simulink model "hyun_PotensionMetor_To_Dcmotor"  (R2022b)
settings: Solver=ode4  StartTime=0.0  StopTime=inf  RelTol=1e-3  EnableMultiTasking=on
libraries: arduinolib x3
settings Model: ExtModeTrigDuration=2  Creator=user  LastModifiedBy=현대오토18
settings OptimizationCC: EnhancedBackFolding=on  PassReuseOutputArgsAs=Individual arguments  ZeroExternalMemoryAtStartup=off  ZeroInternalMemoryAtStartup=off  MaxStackSize=64  OptimizeBlockOrder=speed  DifferentSizesBufferReuse=on  OptimizationCustomize=off  EfficientTunableParamExpr=on
settings DebuggingCC: ParameterTunabilityLossMsg=error
settings HardwareCC: ProdBitPerInt=16  ProdBitPerPointer=16  ProdBitPerSizeT=16  ProdBitPerPtrDiffT=16  ProdLargestAtomicFloat=None  ProdWordSize=8  ProdHWDeviceType=Atmel->AVR
settings SFSimCC: MATLABDynamicMemAlloc=off
settings RTWCC: Description=Embedded Coder  SystemTargetFile=ert.tlc  HardwareBoard=Arduino Mega 2560  TLCOptions=-aInlineSetEventsForThisBaseRateFcn=TLC_FALSE -aSuppressMultiTaskScheduler=TLC_FALSE -aRateBasedStepFcn=1  TemplateMakefile=ert_default_tmf  Toolchain=Arduino AVR  BuildConfiguration=Faster Runs
settings CodeAppCC: ForceParamTrailComments=on  IgnoreCustomStorageClasses=off  OperatorAnnotations=on  SimulinkDataObjDesc=on  SFDataObjDesc=on  InsertBlockDesc=on
settings ERTTargetCC: SupportContinuousTime=on  SupportVariableSizeSignals=on  ExtModeTransport=3  ExtModeStaticAlloc=on  ExtModeAutomaticAllocSize=off  ExtModeStaticAllocSize=2048  ExtModeMexFile=ext_xcp  ExtModeIntrfLevel=Level2 - Open

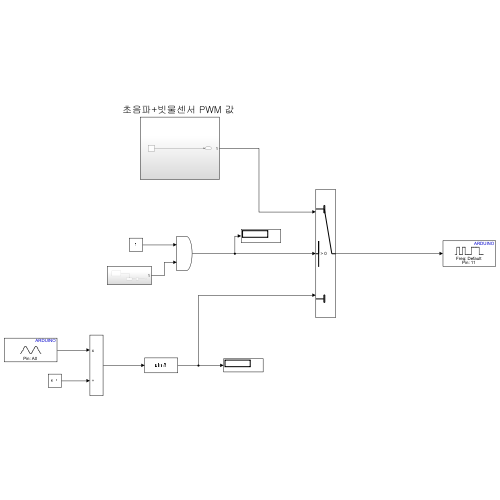
[thumbnail: Simulink's stored preview of the top-level diagram]
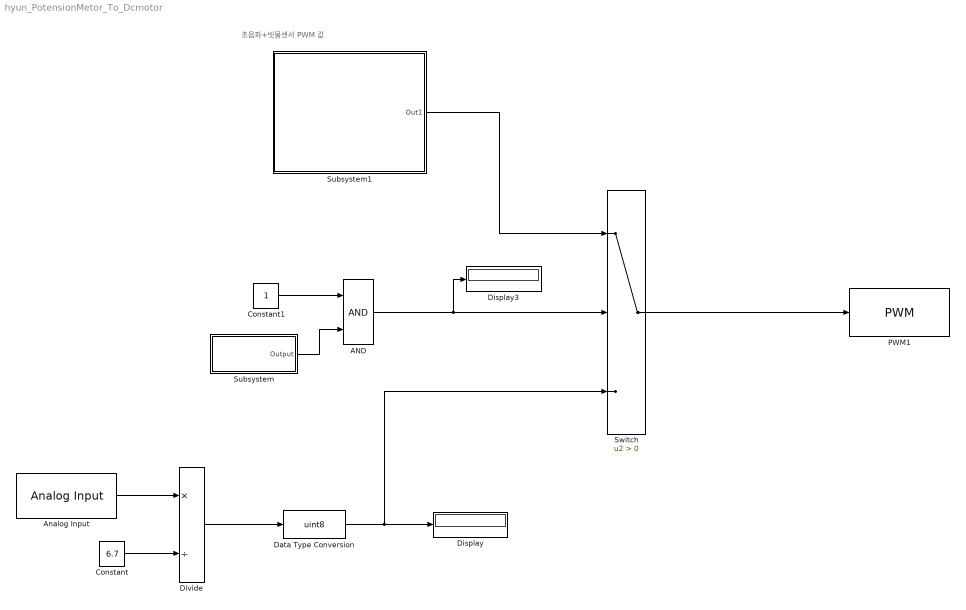
== system hyun_PotensionMetor_To_Dcmotor ==
  note: 초음파+빗물센서 PWM 값
  AND : Logic  IconShape=distinctive  AllPortsSameDT=off  OutDataTypeStr=boolean
  Analog Input : arduinolib/Analog Input  pinNumber=0  ReadResultsOnly=off  ConversionTriggerSource=Software  ExternalTriggerType=uint32( 0 )  OutputDataType=uint16  EnableConversionCompleteNotify=off  EnableOuputStatus=off  SampleTime=-1  blockPlatform=arduino
  Constant : Constant  Value=6.7
  Constant1 : Constant
  Data Type Conversion : DataTypeConversion  OutDataTypeStr=uint8  SaturateOnIntegerOverflow=off  RndMeth=Floor
  Display : Display
  Display3 : Display
  Divide : Product  Inputs=*/
  PWM1 : arduinolib/PWM  pinNumber=11  frequencyType=Default  desiredFrequency=490.2  achievableFrequency=490.2
  Subsystem : Subsystem
  Subsystem1 : Subsystem
  Switch : Switch  Criteria=u2 > Threshold  SaturateOnIntegerOverflow=off  InputSameDT=off
  wires:
  Divide/1 -> Data Type Conversion/1
  AND/1 -> Display3/1, Switch/2
  Constant/1 -> Divide/2
  Data Type Conversion/1 -> Switch/3, Display/1
  Constant1/1 -> AND/1
  Analog Input/1 -> Divide/1
  Subsystem/1(Output) -> AND/2
  Switch/1 -> PWM1/1
  Subsystem1/1(Out1) -> Switch/1

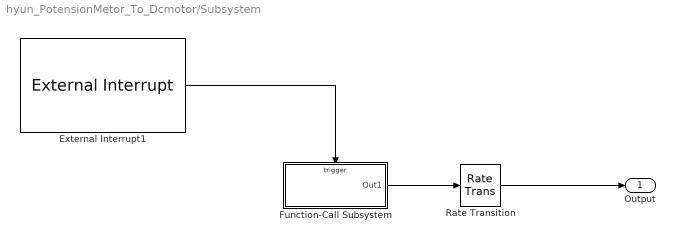
== system hyun_PotensionMetor_To_Dcmotor/Subsystem ==
  External Interrupt1 : arduinolib/External Interrupt  Pin=2  PullUp=off  Mode=FALLING  InterruptSimulationInput=off
  Function-Call Subsystem : Subsystem  TreatAsAtomicUnit=on
  Rate Transition : RateTransition  Deterministic=off
  Output : Outport
  wires:
  Function-Call Subsystem/1(Out1) -> Rate Transition/1
  External Interrupt1/1 -> Function-Call Subsystem/Trigger
  Rate Transition/1 -> Output/1

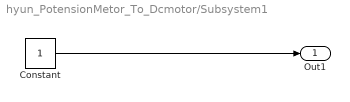
== system hyun_PotensionMetor_To_Dcmotor/Subsystem1 ==
  Constant : Constant
  Out1 : Outport
  wires:
  Constant/1 -> Out1/1

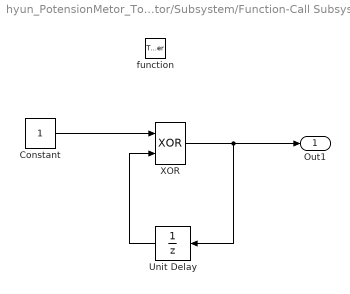
== system hyun_PotensionMetor_To_Dcmotor/Subsystem/Function-Call Subsystem ==
  function : TriggerPort  TriggerType=function-call  VariantControl=(inherit)
  Constant : Constant
  Unit Delay : UnitDelay  InitialCondition=1  SampleTime=-1  HasFrameUpgradeWarning=on
  XOR : Logic  Operator=XOR  IconShape=distinctive  AllPortsSameDT=off  OutDataTypeStr=boolean
  Out1 : Outport
  wires:
  Constant/1 -> XOR/1
  XOR/1 -> Unit Delay/1, Out1/1
  Unit Delay/1 -> XOR/2
